simulink model "simulasi"  (R2016a)
settings: Solver=VariableStepAuto  StartTime=0.0  StopTime=5  RelTol=1e-3
settings Model: Creator=Asus  LastModifiedBy=krishna

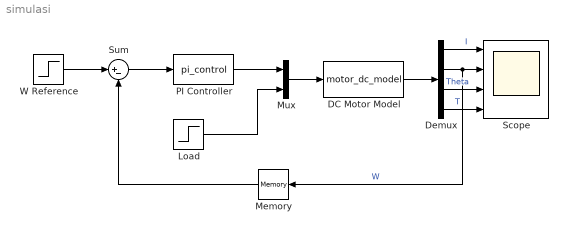
== system simulasi ==
  DC Motor Model : S-Function  FunctionName=motor_dc_model  SFunctionDeploymentMode=off  EnableBusSupport=off
  Demux : Demux
  Load : Step  Time=0  After=2  SampleTime=0
  Memory : Memory
  Mux : Mux  Inputs=2
  PI Controller : S-Function  FunctionName=pi_control  SFunctionDeploymentMode=off  EnableBusSupport=off
  Scope : Scope  NumInputPorts=4
  Sum : Sum  Inputs=|+-
  W Reference : Step  Time=0  After=14  SampleTime=0
  wires:
  W Reference/1 -> Sum/1
  Sum/1 -> PI Controller/1
  PI Controller/1 -> Mux/1
  DC Motor Model/1 -> Demux/1
  Demux/2 -> Memory/1, Scope/2  "W"
  Demux/1 -> Scope/1  "I"
  Demux/3 -> Scope/3  "Theta"
  Demux/4 -> Scope/4  "T"
  Memory/1 -> Sum/2
  Load/1 -> Mux/2
  Mux/1 -> DC Motor Model/1
